simulink model "FIR_InterpolationStream_Ex3"  (R2024a)
settings: Solver=VariableStepAuto  StartTime=0.0  StopTime=10.0  RelTol=1e-3
InitFcn:
  | Fs = 50e3;               % Sampling Frequency
  | Fpass = 16000;            % Passband Frequency
  | Fstop = 23000;            % Stopband Frequency
  | Dpass = 0.00460513763;    % Passband Ripple
  | Dstop = 0.0001;           % Stopband Attenuation
  | dens  = 16;                   % Density Factor
  | % Calculate the order from the parameters using FIRPMORD.
  | [N, Fo, Ao, W] = firpmord([Fpass, Fstop]/(Fs/2), [1 0], [Dpass, Dstop]);
  | % Calculate the coefficients using the FIRPM function.
  | b  = firpm(N, Fo, Ao, W, {dens});
  | coeffs = b;
undefined symbols (not defined in the file): None, S, vsva2197, xcvc1902
libraries: aieUtilities x2, dspsrcs4 x1, aieDSP x1, dspmlti4 x1, vmcUtilities x1
settings Model: Creator=sdegala  LastModifiedBy=robg
settings DebuggingCC: UnderspecifiedInitializationDetection=Classic  MergeDetectMultiDrivingBlocksExec=none
settings ModelReferenceCC: PropagateSignalLabelsOutOfModel=off

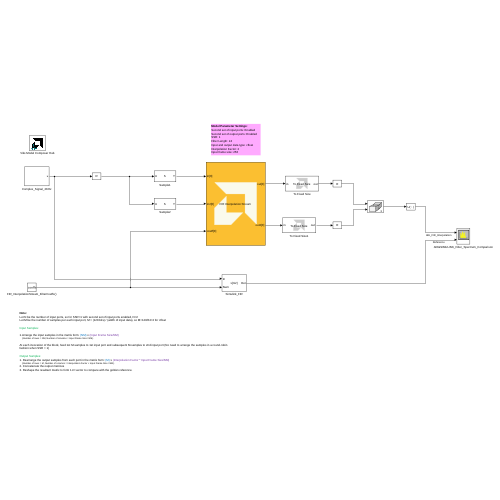
[thumbnail: Simulink's stored preview of the top-level diagram]
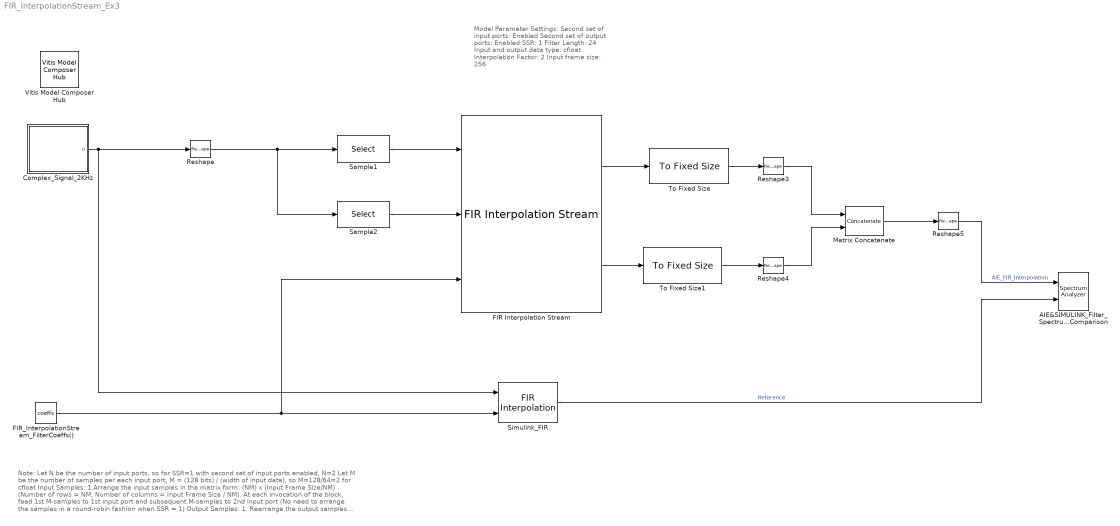
== system FIR_InterpolationStream_Ex3 ==
  note: Note:
      | Let N be the number of input ports, so for SSR=1 with second set of input ports enabled, N=2
      | Let M be the number of samples per each input port, M = (128 bits) / (width of input data), so M=128/64=2 for cfloat
      |
      | Input Samples:
      |
      | 1.Arrange the input samples in the matrix form: (NM) x (Input Frame Size/NM)
      | (Number of rows = NM, Number of columns = Input Frame Size / NM).
      |
      | At each invocation of the block, feed 1st M-samples to 1st input port and subsequent M-samples to 2nd input port (No need to arrange the samples in a round-robin fashion when SSR = 1)
      |
      | Output Samples:
      | 1. Rearrange the output samples from each port in the matrix form: (M) x (Interpolation Factor * Input Frame Size/NM)
      | (Number of rows = M, Number of columns = Interpolation Factor × Input Frame Size / NM).
      | 2. Concatenate the output matrices
      | 3. Reshape the resultant matrix to form 1-D vector to compare with the golden reference.
  note: Model Parameter Settings:
      | Second set of input ports: Enabled
      | Second set of output ports: Enabled
      | SSR: 1
      | Filter Length: 24
      | Input and output data type: cfloat
      | Interpolation Factor: 2
      | Input frame size: 256
  AIE&SIMULINK_Filter_Spectrum_Comparison : SpectrumAnalyzer  NumInputPorts=2  WindowPosition=[771.000000,408.000000,800.000000,500.000000,]  Visible=on  ScopeFrameLocation=window  Span=49999.99999999999  StartFrequency=-24999.999999999996  StopFrequency=24999.999999999996  AveragingMethod=Exponential  YLimits=[-85.1987 36.07]  ShowLegend=on  ChannelNames="[\"\"]"  AllowFFTLengthLessThanSamplesPerUpdate=on  DefaultConfigurationName=spbscopes.SpectrumAnalyzerBlockCfg
  Complex_Signal_2KHz : Subsystem
  FIR Interpolation Stream : aieDSP/FIR Interpolation Stream  data_type=cfloat  coef_type=float  use_coeff_reload=on  dual_ip=on  num_outputs=on  coeff=coeffs  fir_length=24  interpolate_factor=2  input_window_size=256  shift_val=0  rnd_mode=Round to positive infinity  sat_mode=0-None  ssr=1  interp_poly=1  casc_length=1  AIE_VARIANT=1  TP_API=1  blockJsonConstraints=[]  blockJsonConstraintsInternal=[]  spec=vmc_stream_fir_interpolate_asym.json  SerializedMaskParamNames=[]  SerializedMaskParamValues=[]  SerializedMaskParamVisibilities=[]  block_type=FIR Interpolation Stream  SerializedMaskParamDataypes=typename|typename|uint|uint|uint|coef_type|uint|uint|uint|uint|uint|uint|uint|uint|uint|uint|uint  SerializedMaskParamEnumStrArr=0|0|0|0|0|0|0|0|0|0|Floor,Ceiling,Round to positive infinity,Round to negative infinity,Round symmetrical to infinity,Round symmetrical to zero,Round convergent to even,Round convergent to odd|0-None,1-Asymmetric,3-Symmetric|0|0|0|0|0  SerializedMaskParamEnumValArr=0|0|0|0|0|0|0|0|0|0|0,1,2,3,4,5,6,7|0,1,3|0|0|0|0|0  SerializedMaskParamVectorArr=0|0|0|0|0|1|0|0|0|0|0|0|0|0|0|0|0  SerializedMaskParamKeys=TT_DATA|TT_COEFF|TP_USE_COEFF_RELOAD|TP_DUAL_IP|TP_NUM_OUTPUTS|coeff|TP_FIR_LEN|TP_INTERPOLATE_FACTOR|TP_INPUT_WINDOW_VSIZE|TP_SHIFT|TP_RND|TP_SAT|TP_SSR|TP_PARA_INTERP_POLY|TP_CASC_LEN|AIE_VARIANT|TP_API
  FIR_InterpolationStream_FilterCoeffs() : Constant  Value=coeffs  OutDataTypeStr=single
  Matrix Concatenate : Concatenate  Mode=Multidimensional array
  Reshape : Reshape  OutputDimensionality=Customize  OutputDimensions=[4,64]
  Reshape3 : Reshape  OutputDimensionality=Customize  OutputDimensions=[2,128]
  Reshape4 : Reshape  OutputDimensionality=Customize  OutputDimensions=[2,128]
  Reshape5 : Reshape
  Sample1 : Selector  NumberOfDimensions=2  InputPortWidth=256  IndexOptions=Index vector (dialog),Select all  Indices=[1 2],1  OutputSizes=1,1
  Sample2 : Selector  NumberOfDimensions=2  InputPortWidth=256  IndexOptions=Index vector (dialog),Select all  Indices=[3 4],1  OutputSizes=1,1
  "Simulink_FIR " : dspmlti4/FIR Interpolation  FilterSource=Input port  PrivateCoeffs=0  h=coeffs  L=2  FilterObject=FINTERP  InputProcessing=Columns as channels (frame based)  framing=Enforce single-rate processing  outputBufInitCond=0  roundingMode=Ceiling  overflowMode=off  firstCoeffDataTypeStr=Inherit: Same word length as input  firstCoeffMin=[]  firstCoeffMax=[]  firstCoeffLastDataTypeStr=Inherit: Same word length as input  outputMin=[]  outputMax=[]
  To Fixed Size : aieUtilities/To Fixed Size  Mode=Stop simulation when input variable-size signal is not full  OutputSize=Inherit: Same as input  CopyMethod=Buffer samples to form output  HasStatusOutput=on
  To Fixed Size1 : aieUtilities/To Fixed Size  Mode=Stop simulation when input variable-size signal is not full  OutputSize=Inherit: Same as input  CopyMethod=Buffer samples to form output  HasStatusOutput=on
  Vitis Model Composer Hub : vmcUtilities/Vitis Model Composer Hub  Tag=genX  CodeGeneration=off  StartColumn=1  NumberOfColumns=1  TargetDirectory=./code  exportDesign=off  analyzeDesign=off  validateDesignOnHw=off  ExportType=AI Engines  IpVendor=xilinx.com  IpLibrary=hls  IpVersion=1.0  IpHWLanguage=Verilog  AieCompilerOptions={}  AieSimulatorOptions={}  CreateTestbench=off  TestbenchStackSize=10  RunRtlSim=off  RunCSim=off  RunAieSim=off  AieSimTimeout=50000  RunAieSimProfiling=off  LaunchVitisAnalyzer=off  PlotOutput=off  RunX86Sim=off  X86SimTimeout=10  GenHwImage=off  GenLibadfXo=off  GenHwValidationCode=off  PlatformType=Not Specified  HwSystemType=Baremetal  HwValidationTarget=hw  ProjDevice=xcvc1902-vsva2197-1LP-e-S  ProjDevicePart=xcvc1902-vsva2197-1LP-e-S  AIEType=AIE  SamplePeriod=-1  ClockFrequency=200  DataPathParallelism=1  xilinxfamily=versalaicore  part=xcvc1902  speed=-1LP-e-S  package=vsva2197  directory=./netlist  testbench=off  incr_netlist=off  synthesis_tool=Vivado  clock_wrapper=Clock Enables  dbl_ovrd=According to Block Masks  dcm_input_clock_period=10  sysclk_period=10  simulink_period=1  eval_field=0  LogFileName=''  NThreads=4
  wires:
  FIR_InterpolationStream_FilterCoeffs()/1 -> "Simulink_FIR "/2, FIR Interpolation Stream/3
  Complex_Signal_2KHz/1(u) -> "Simulink_FIR "/1, Reshape/1
  "Simulink_FIR "/1 -> AIE&SIMULINK_Filter_Spectrum_Comparison/2  "Reference"
  FIR Interpolation Stream/1 -> To Fixed Size/1
  FIR Interpolation Stream/2 -> To Fixed Size1/1
  To Fixed Size/1 -> Reshape3/1
  To Fixed Size1/1 -> Reshape4/1
  Matrix Concatenate/1 -> Reshape5/1
  Reshape/1 -> Sample2/1, Sample1/1
  Sample1/1 -> FIR Interpolation Stream/1
  Sample2/1 -> FIR Interpolation Stream/2
  Reshape3/1 -> Matrix Concatenate/1
  Reshape4/1 -> Matrix Concatenate/2
  Reshape5/1 -> AIE&SIMULINK_Filter_Spectrum_Comparison/1  "AIE_FIR_Interpolation"

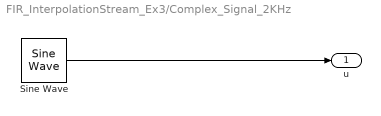
== system FIR_InterpolationStream_Ex3/Complex_Signal_2KHz ==
  Sine Wave : dspsrcs4/Sine Wave  Amplitude=1  Frequency=2e3  Phase=0  SampleMode=Discrete  OutComplex=Complex  CompMethod=Trigonometric fcn  TableSize=Speed  SampleTime=1/25e3  SamplesPerFrame=256  ResetState=Restart at time zero  OutputFrames=off  dataType=single  wordLen=16  udDataType=sfix(16)  fracBitsMode=Best precision  numFracBits=15  OutDataTypeStr=single  LastOutDataTypeStr=single
  u : Outport
  wires:
  Sine Wave/1 -> u/1
